simulink model "etc_throttle"  (R2018a)
settings: Solver=ode45  StartTime=0.0  StopTime=20.0  RelTol=1e-3  EnableMultiTasking=on
PreLoadFcn:
  | etc_plant_data;
values from neighbouring files (symbols this model uses):
  J = 0.000245    [allParamValues.mat]
Description:
  | This is my help
settings Model: ParamWorkspaceSource=ReferencedWorkspace  Creator=koliver  LastModifiedBy=bneiswan
settings DataIOCC: ExternalInput=[t, duty, direction]  LimitDataPoints=on  LoadExternalInput=on  SaveFormat=Array  SignalLoggingName=sigsOut
settings OptimizationCC: DefaultParameterBehavior=Inlined  ExpressionDepthLimit=2147483647  InitFltsAndDblsToZero=on  LifeSpan=inf
settings DebuggingCC: SaveWithParameterizedLinksMsg=none  UnderspecifiedInitializationDetection=Classic  MergeDetectMultiDrivingBlocksExec=none  MultiTaskDSMMsg=warning  MultiTaskCondExecSysMsg=none  ParameterPrecisionLossMsg=none  FcnCallInpInsideContextMsg=warning  AllowSymbolicDim=off  StateNameClashWarn=warning  SFUnexpectedBacktrackingDiag=warning  SFNoUnconditionalDefaultTransitionDiag=warning  SFExecutionAtInitializationDiag=none
settings HardwareCC: ProdBitPerPointer=32  ProdBitPerSizeT=32  ProdBitPerPtrDiffT=32  ProdLargestAtomicFloat=None  ProdIntDivRoundTo=Undefined  ProdEndianess=Unspecified  ProdWordSize=32  ProdHWDeviceType=32-bit Generic  TargetIntDivRoundTo=Zero  TargetEndianess=BigEndian  TargetHWDeviceType=Motorola PowerPC
settings ModelReferenceCC: ModelReferenceNumInstancesAllowed=Single  PropagateSignalLabelsOutOfModel=off
settings SFSimCC: SimParseCustomCode=off
settings CodeAppCC: StateflowObjectComments=on
settings GRTTargetCC: TargetFcnLib=ansi_tfl_tmw.mat  TargetLangStandard=C89/C90 (ANSI)  GeneratePreprocessorConditionals=Disable all  CombineOutputUpdateFcns=off  GRTInterface=on
settings ConfigComp: CovMetricSettings=dw  CovHtmlReporting=on  CovSaveCumulativeToWorkspaceVar=on  CovSaveSingleToWorkspaceVar=on  CovExternalEMLEnable=off  CovSFcnEnable=off

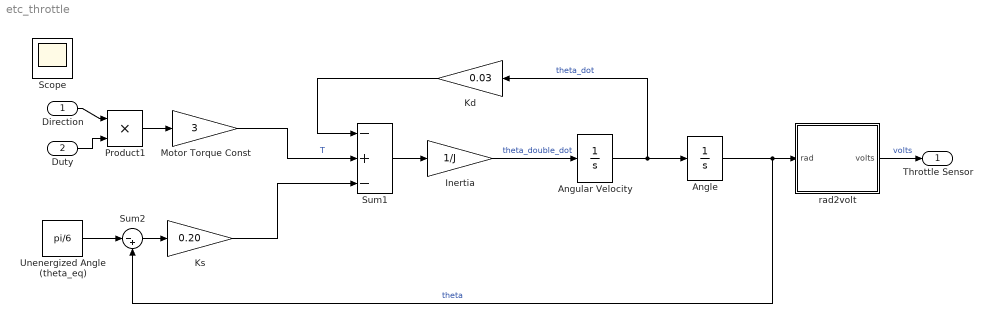
== system etc_throttle ==
  Direction : Inport
  Duty : Inport  Port=2
  Angle : Integrator  InitialCondition=pi/6  LimitOutput=on  UpperSaturationLimit=pi/2  LowerSaturationLimit=0
      settings: AttributesFormatString=%<LowerSaturationLimit> <= th <= %<UpperSaturationLimit>
  Angular Velocity : Integrator
  Inertia : Gain  Gain=1/J  SaturateOnIntegerOverflow=on  OutDataTypeStr=Inherit: Same as input  ParamDataTypeStr=Inherit: Same as input
  Kd : Gain  Gain=0.03  SaturateOnIntegerOverflow=on  OutDataTypeStr=Inherit: Same as input  ParamDataTypeStr=Inherit: Same as input
  Ks : Gain  Gain=0.20  SaturateOnIntegerOverflow=on  OutDataTypeStr=Inherit: Same as input  ParamDataTypeStr=Inherit: Same as input
  Motor Torque Const : Gain  Gain=3  SaturateOnIntegerOverflow=on  OutDataTypeStr=Inherit: Same as input  ParamDataTypeStr=Inherit: Same as input
  Product1 : Product  SaturateOnIntegerOverflow=on  OutDataTypeStr=Inherit: Same as first input
  Sum1 : Sum  Inputs=-+-  SaturateOnIntegerOverflow=on
  Sum2 : Sum  Inputs=|-+  SaturateOnIntegerOverflow=on
  Unenergized Angle (theta_eq) : Constant  Value=pi/6
  rad2volt : Subsystem
  Throttle Sensor : Outport
  Scope : Scope
  wires:
  rad2volt/1(volts) -> Throttle Sensor/1  "volts"
  Product1/1 -> Motor Torque Const/1
  Unenergized Angle (theta_eq)/1 -> Sum2/1
  Sum2/1 -> Ks/1
  Angle/1 -> Sum2/2, rad2volt/1(rad)  "theta"
  Angular Velocity/1 -> Angle/1, Kd/1  "theta_dot"
  Inertia/1 -> Angular Velocity/1  "theta_double_dot"
  Direction/1 -> Product1/1
  Duty/1 -> Product1/2
  Motor Torque Const/1 -> Sum1/2  "T"
  Kd/1 -> Sum1/1
  Ks/1 -> Sum1/3
  Sum1/1 -> Inertia/1

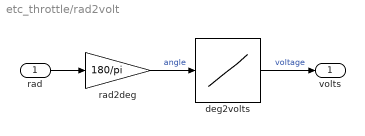
== system etc_throttle/rad2volt ==
  rad : Inport
  deg2volts : Lookup_n-D  NumberOfTableDimensions=1  BreakpointsForDimension1=[0 90]  Table=[0.5 4.5]  RndMeth=Simplest  InputSameDT=on
  rad2deg : Gain  Gain=180/pi  SaturateOnIntegerOverflow=on  OutDataTypeStr=Inherit: Same as input  ParamDataTypeStr=Inherit: Same as input
  volts : Outport
  wires:
  deg2volts/1 -> volts/1  "voltage"
  rad/1 -> rad2deg/1
  rad2deg/1 -> deg2volts/1  "angle"
